simulink model "nh"  (R2021b)
settings: Solver=VariableStepAuto  StartTime=0.0  StopTime=25  RelTol=1e-10
values from neighbouring files (symbols this model uses):
  R = 1    [main.m]
  wd = 0.5    [main.m]
  x0 = [x20; x30 + x20 * b_0 * T]    [nakamura.m]
undefined symbols (not defined in the file or in its folder): K1, K2, o0, y0
settings Model: Creator=mbober  LastModifiedBy=mbober

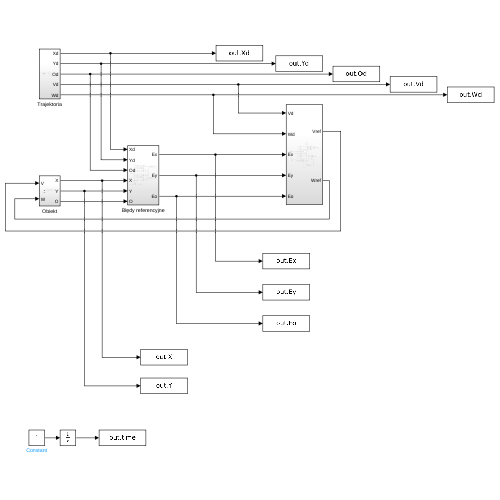
[thumbnail: Simulink's stored preview of the top-level diagram]
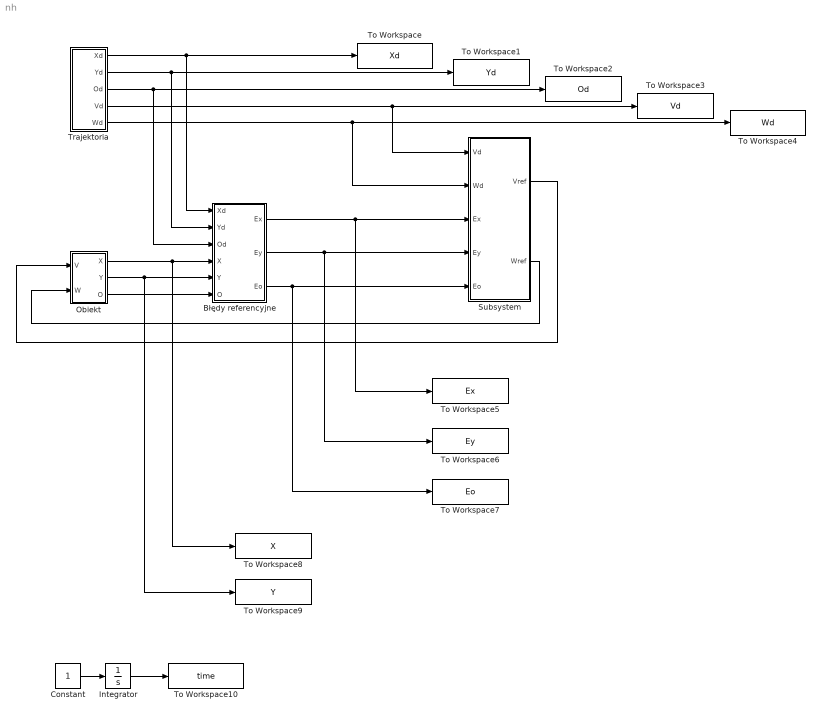
== system nh ==
  Błędy referencyjne : Subsystem
  Constant : Constant
  Integrator : Integrator
  Obiekt : Subsystem
  Subsystem : Subsystem
  To Workspace : ToWorkspace  VariableName=Xd  SampleTime=-1
  To Workspace1 : ToWorkspace  VariableName=Yd  SampleTime=-1
  To Workspace10 : ToWorkspace  VariableName=time  SampleTime=-1
  To Workspace2 : ToWorkspace  VariableName=Od  SampleTime=-1
  To Workspace3 : ToWorkspace  VariableName=Vd  SampleTime=-1
  To Workspace4 : ToWorkspace  VariableName=Wd  SampleTime=-1
  To Workspace5 : ToWorkspace  VariableName=Ex  SampleTime=-1
  To Workspace6 : ToWorkspace  VariableName=Ey  SampleTime=-1
  To Workspace7 : ToWorkspace  VariableName=Eo  SampleTime=-1
  To Workspace8 : ToWorkspace  VariableName=X  SampleTime=-1
  To Workspace9 : ToWorkspace  VariableName=Y  SampleTime=-1
  Trajektoria : Subsystem
  wires:
  Trajektoria/1(Xd) -> Błędy referencyjne/1(Xd), To Workspace/1
  Trajektoria/2(Yd) -> Błędy referencyjne/2(Yd), To Workspace1/1
  Trajektoria/3(Od) -> Błędy referencyjne/3(Od), To Workspace2/1
  Trajektoria/4(Vd) -> Subsystem/1(Vd), To Workspace3/1
  Trajektoria/5(Wd) -> Subsystem/2(Wd), To Workspace4/1
  Obiekt/1(X) -> To Workspace8/1, Błędy referencyjne/4(X)
  Obiekt/2(Y) -> To Workspace9/1, Błędy referencyjne/5(Y)
  Obiekt/3(O) -> Błędy referencyjne/6(O)
  Błędy referencyjne/1(Ex) -> To Workspace5/1, Subsystem/3(Ex)
  Błędy referencyjne/2(Ey) -> To Workspace6/1, Subsystem/4(Ey)
  Błędy referencyjne/3(Eo) -> To Workspace7/1, Subsystem/5(Eo)
  Subsystem/1(Vref) -> Obiekt/1(V)
  Subsystem/2(Wref) -> Obiekt/2(W)
  Constant/1 -> Integrator/1
  Integrator/1 -> To Workspace10/1

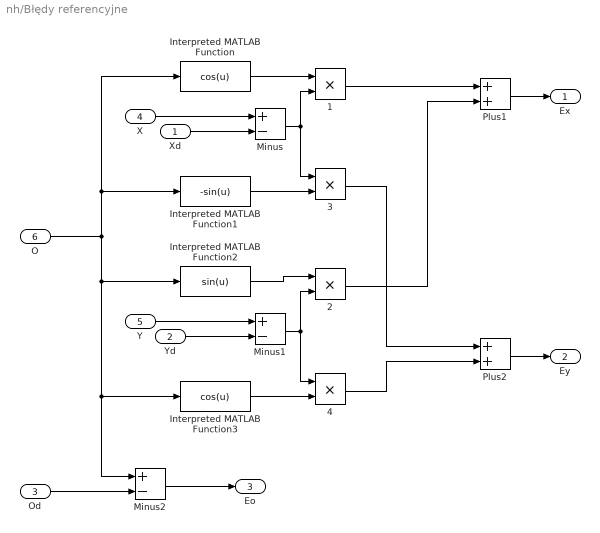
== system nh/Błędy referencyjne ==
  Xd : Inport
  Yd : Inport  Port=2
  Od : Inport  Port=3
  X : Inport  Port=4
  Y : Inport  Port=5
  O : Inport  Port=6
  {1..4} (4 alike) : Product
  Interpreted MATLAB Function : MATLABFcn  MATLABFcn=cos(u)
  Interpreted MATLAB Function1 : MATLABFcn  MATLABFcn=-sin(u)
  Interpreted MATLAB Function2 : MATLABFcn  MATLABFcn=sin(u)
  Interpreted MATLAB Function3 : MATLABFcn  MATLABFcn=cos(u)
  Minus : Sum  Inputs=+-
  Minus1 : Sum  Inputs=+-
  Minus2 : Sum  Inputs=+-
  Plus1 : Sum
  Plus2 : Sum
  Ex : Outport
  Ey : Outport  Port=2
  Eo : Outport  Port=3
  wires:
  Plus1/1 -> Ex/1
  Minus/1 -> 3/1, 1/2
  O/1 -> Interpreted MATLAB Function/1, Interpreted MATLAB Function1/1, Minus2/1, Interpreted MATLAB Function3/1, Interpreted MATLAB Function2/1
  Od/1 -> Minus2/2
  Interpreted MATLAB Function3/1 -> 4/2
  Yd/1 -> Minus1/2
  Minus1/1 -> 4/1, 2/2
  Plus2/1 -> Ey/1
  2/1 -> Plus1/2
  1/1 -> Plus1/1
  Interpreted MATLAB Function1/1 -> 3/2
  4/1 -> Plus2/2
  Interpreted MATLAB Function2/1 -> 2/1
  Xd/1 -> Minus/2
  Minus2/1 -> Eo/1
  X/1 -> Minus/1
  3/1 -> Plus2/1
  Interpreted MATLAB Function/1 -> 1/1
  Y/1 -> Minus1/1

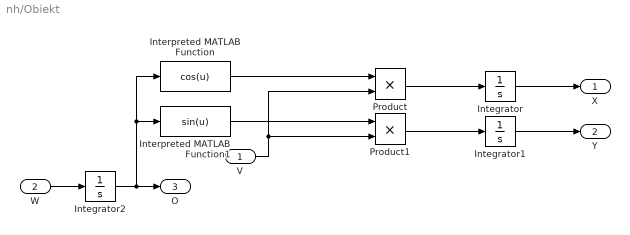
== system nh/Obiekt ==
  V : Inport
  W : Inport  Port=2
  Integrator : Integrator  InitialCondition=x0
  Integrator1 : Integrator  InitialCondition=y0
  Integrator2 : Integrator  InitialCondition=o0
  Interpreted MATLAB Function : MATLABFcn  MATLABFcn=cos(u)
  Interpreted MATLAB Function1 : MATLABFcn  MATLABFcn=sin(u)
  Product : Product
  Product1 : Product
  X : Outport
  Y : Outport  Port=2
  O : Outport  Port=3
  wires:
  Product1/1 -> Integrator1/1
  Product/1 -> Integrator/1
  Integrator/1 -> X/1
  Integrator2/1 -> O/1, Interpreted MATLAB Function/1, Interpreted MATLAB Function1/1
  V/1 -> Product1/2, Product/2
  Integrator1/1 -> Y/1
  Interpreted MATLAB Function1/1 -> Product1/1
  W/1 -> Integrator2/1
  Interpreted MATLAB Function/1 -> Product/1

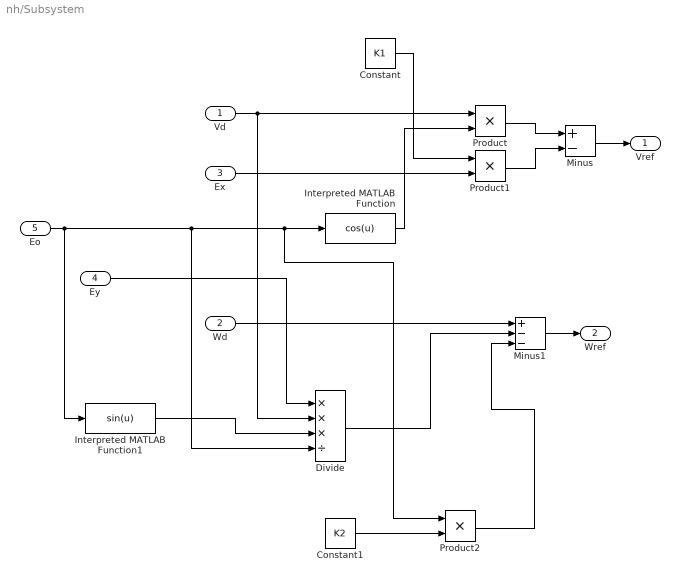
== system nh/Subsystem ==
  Vd : Inport
  Wd : Inport  Port=2
  Ex : Inport  Port=3
  Ey : Inport  Port=4
  Eo : Inport  Port=5
  Constant : Constant  Value=K1
  Constant1 : Constant  Value=K2
  Divide : Product  Inputs=***/
  Interpreted MATLAB Function : MATLABFcn  MATLABFcn=cos(u)
  Interpreted MATLAB Function1 : MATLABFcn  MATLABFcn=sin(u)
  Minus : Sum  Inputs=+-
  Minus1 : Sum  Inputs=+--
  Product : Product
  Product1 : Product
  Product2 : Product
  Vref : Outport
  Wref : Outport  Port=2
  wires:
  Ex/1 -> Product1/2
  Divide/1 -> Minus1/2
  Ey/1 -> Divide/1
  Constant1/1 -> Product2/2
  Vd/1 -> Divide/2, Product/1
  Minus/1 -> Vref/1
  Eo/1 -> Interpreted MATLAB Function1/1, Divide/4, Product2/1, Interpreted MATLAB Function/1
  Minus1/1 -> Wref/1
  Wd/1 -> Minus1/1
  Interpreted MATLAB Function1/1 -> Divide/3
  Interpreted MATLAB Function/1 -> Product/2
  Product2/1 -> Minus1/3
  Product1/1 -> Minus/2
  Product/1 -> Minus/1
  Constant/1 -> Product1/1

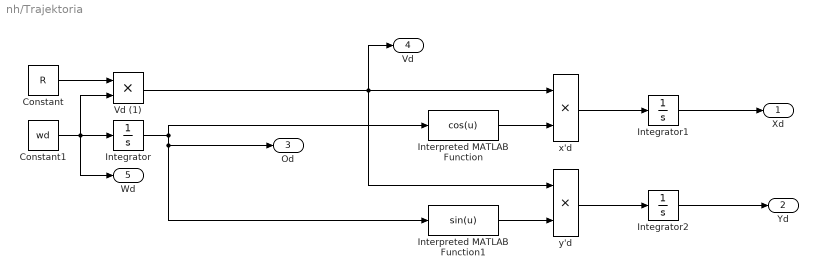
== system nh/Trajektoria ==
  Constant : Constant  Value=R
  Constant1 : Constant  Value=wd
  Integrator : Integrator
  Integrator1 : Integrator
  Integrator2 : Integrator  InitialCondition=-R
  Interpreted MATLAB Function : MATLABFcn  MATLABFcn=cos(u)
  Interpreted MATLAB Function1 : MATLABFcn  MATLABFcn=sin(u)
  Vd (1) : Product
  x'd : Product
  y'd : Product
  Xd : Outport
  Yd : Outport  Port=2
  Od : Outport  Port=3
  Vd : Outport  Port=4
  Wd : Outport  Port=5
  wires:
  y'd/1 -> Integrator2/1
  Interpreted MATLAB Function/1 -> x'd/2
  Integrator1/1 -> Xd/1
  Constant/1 -> Vd (1)/1
  Integrator2/1 -> Yd/1
  Constant1/1 -> Wd/1, Vd (1)/2, Integrator/1
  Integrator/1 -> Od/1, Interpreted MATLAB Function1/1, Interpreted MATLAB Function/1
  x'd/1 -> Integrator1/1
  Vd (1)/1 -> Vd/1, y'd/1, x'd/1
  Interpreted MATLAB Function1/1 -> y'd/2
